simulink model "Citation"  (Simulink 10.0)
settings: Solver=ode5  StartTime=0.0  StopTime=700  FixedStep=0.01  RelTol=1e-3  EnableMultiTasking=on
values from neighbouring files (symbols this model uses):
  x0 = []    [cessnac550_3d_sfnc.m]
undefined symbols (not defined in the file or in its folder): chord, cv1, cv2, cv3, cv4, deltagmax1, deltagmax2, deltagmax3, deltagmax4, Deng, ealphag, ealphas, g0, hDME, hGS, kt1, kt2, kt3, lh, massinit, matbuaf, matdaf, matdam, matdbbf, matdeaf, matdgaf, matdqaf, matduaf, matdwaw, matedhr, mateif, matelhr, matemhr, matemv1, matemv2, matemve, matetam, mateuaf, matfaaf, matfaxl, matff, matibaf, matibmh, matipaf, matipmh, matiraf, matiuaf, matiwaf, matlaf, matlam, matleaf, matleam, matlgaf, matlqaf, matluaf, matmaaf, matmaam, matmaf, matmam, matmbbf ... (+77)
undefined symbols (not defined in the file): matibb
libraries: simulink x8, vrlib x1
(part 5 of 5)

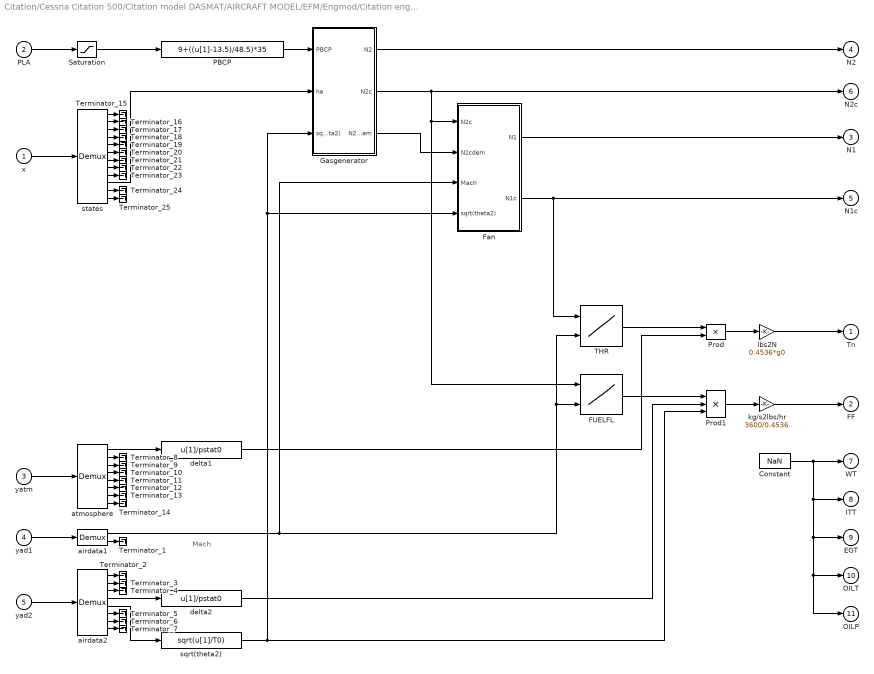
== system Citation/Cessna Citation 500/Citation model DASMAT/AIRCRAFT MODEL/EFM/Engmod/Citation eng_mod/Subsystem1/JT15 Dynamic1/Subsystem/engine ==
  note: Mach
  x : Inport
  PLA : Inport  Port=2
  yatm : Inport  Port=3
  yad1 : Inport  Port=4
  yad2 : Inport  Port=5
  Constant : Constant  Value=NaN
  FUELFL : Lookup2D  RowIndex=matff(2:14,1)  ColumnIndex=matff(1,2:14)  Table=matff(2:14,2:14)  SaturateOnIntegerOverflow=on  InputSameDT=on
  Fan : Subsystem
  Gasgenerator : Subsystem
  PBCP : Fcn  Expr=9+((u[1]-13.5)/48.5)*35
  Prod : Product  SaturateOnIntegerOverflow=on  InputSameDT=on  OutDataTypeStr=Inherit: Same as first input
  Prod1 : Product  Inputs=3  SaturateOnIntegerOverflow=on  InputSameDT=on  OutDataTypeStr=Inherit: Same as first input
  Saturation : Saturate  UpperLimit=62  LowerLimit=13.5
  THR : Lookup2D  RowIndex=matthr(2:12,1)  ColumnIndex=matthr(1,2:12)  Table=matthr(2:12,2:12)  SaturateOnIntegerOverflow=on  InputSameDT=on
  Terminator_{1..25} (25 alike) : Terminator
  airdata1 : Demux  Outputs=2
  airdata2 : Demux  Outputs=8
  atmosphere : Demux  Outputs=8
  delta1 : Fcn  Expr=u[1]/pstat0
  delta2 : Fcn  Expr=u[1]/pstat0
  kg/s2lbs/hr : Gain  Gain=3600/0.4536  SaturateOnIntegerOverflow=on  OutDataTypeStr=Inherit: Same as input  ParamDataTypeStr=Inherit: Same as input
  lbs2N : Gain  Gain=0.4536*g0  SaturateOnIntegerOverflow=on  OutDataTypeStr=Inherit: Same as input  ParamDataTypeStr=Inherit: Same as input
  sqrt(theta2) : Fcn  Expr=sqrt(u[1]/T0)
  states : Demux  Outputs=12
  Tn : Outport
  FF : Outport  Port=2
  N1 : Outport  Port=3
  N2 : Outport  Port=4
  N1c : Outport  Port=5
  N2c : Outport  Port=6
  WT : Outport  Port=7
  ITT : Outport  Port=8
  EGT : Outport  Port=9
  OILT : Outport  Port=10
  OILP : Outport  Port=11
  wires:
  states/12 -> Terminator_25/1
  states/11 -> Terminator_24/1
  states/9 -> Terminator_23/1
  states/8 -> Terminator_22/1
  states/7 -> Terminator_21/1
  states/6 -> Terminator_20/1
  states/5 -> Terminator_19/1
  states/4 -> Terminator_18/1
  states/3 -> Terminator_17/1
  states/2 -> Terminator_16/1
  states/1 -> Terminator_15/1
  atmosphere/8 -> Terminator_14/1
  atmosphere/7 -> Terminator_13/1
  atmosphere/6 -> Terminator_12/1
  atmosphere/5 -> Terminator_11/1
  atmosphere/4 -> Terminator_10/1
  atmosphere/3 -> Terminator_9/1
  atmosphere/2 -> Terminator_8/1
  airdata2/8 -> Terminator_7/1
  airdata2/7 -> Terminator_6/1
  airdata2/6 -> Terminator_5/1
  airdata2/3 -> Terminator_4/1
  airdata2/2 -> Terminator_3/1
  airdata2/1 -> Terminator_2/1
  airdata1/2 -> Terminator_1/1
  Fan/2(N1c) -> THR/1, N1c/1
  Gasgenerator/2(N2c) -> Fan/1(N2c), FUELFL/1, N2c/1
  Gasgenerator/3(N2cdem) -> Fan/2(N2cdem)
  airdata1/1 -> Fan/3(Mach), FUELFL/2, THR/2
  Fan/1(N1) -> N1/1
  sqrt(theta2)/1 -> Fan/4(sqrt(theta2)), Gasgenerator/3(sqrt(theta2)), Prod1/3
  yad2/1 -> airdata2/1
  yad1/1 -> airdata1/1
  yatm/1 -> atmosphere/1
  airdata2/4 -> delta2/1
  airdata2/5 -> sqrt(theta2)/1
  Constant/1 -> ITT/1, EGT/1, OILT/1, OILP/1, WT/1
  Gasgenerator/1(N2) -> N2/1
  delta1/1 -> Prod/2
  Prod/1 -> lbs2N/1
  THR/1 -> Prod/1
  lbs2N/1 -> Tn/1
  states/10 -> Gasgenerator/2(he)
  delta2/1 -> Prod1/2
  atmosphere/1 -> delta1/1
  Prod1/1 -> kg/s2lbs/hr/1
  kg/s2lbs/hr/1 -> FF/1
  Saturation/1 -> PBCP/1
  PLA/1 -> Saturation/1
  x/1 -> states/1
  PBCP/1 -> Gasgenerator/1(PBCP)
  FUELFL/1 -> Prod1/1

== system Citation/Cessna Citation 500/Citation model DASMAT/AIRCRAFT MODEL/EFM/Engmod/Citation eng_mod/Subsystem1/JT15 Dynamic/Subsystem/engine/Fan ==
  note: N1c feedback
  note: N1cdot
  N2c : Inport
  N2cdem : Inport  Port=2
  Mach : Inport  Port=3
  sqrt(theta2) : Inport  Port=4
  Droop : Gain  Gain=2  SaturateOnIntegerOverflow=on  OutDataTypeStr=Inherit: Same as input  ParamDataTypeStr=Inherit: Same as input
  Max accel : Subsystem  mask(Min Value){}
      mask help:
      | Output is minimum value of inputs.
      | y=min(u1,u2)
      mask Help: The Min block produces as output the minimum value of two scalars or vectors. If the inputs are vectors, the output will be a vector containing the minimum elements of the vectors.
      mask Display: disp('Min')
  Max decel : Subsystem  mask(Max Value){}
      mask help:
      | Output is maximum value of inputs.
      | y=max(u1,u2)
      mask Help: The Max block produces as output the maximum value of two scalars or vectors. If the inputs are vectors, the output will be a vector containing the maximum elements of the vectors.
      mask Display: disp('Max')
  N1 state : Integrator  InitialCondition=xt0(2)
  N1D : Lookup2D  RowIndex=matn1d(2:14,1)  ColumnIndex=matn1d(1,2:14)  Table=matn1d(2:14,2:14)  SaturateOnIntegerOverflow=on  InputSameDT=on
  Prod : Product  SaturateOnIntegerOverflow=on  InputSameDT=on  OutDataTypeStr=Inherit: Same as first input
  Sum : Sum  Inputs=+-  SaturateOnIntegerOverflow=on  InputSameDT=on  OutDataTypeStr=Inherit: Same as first input
  fN1cmax : Lookup  InputValues="[0 25 40 70 94  120]"  Table="[0   0   1   12 14  18]"  SaturateOnIntegerOverflow=on
  fN1cmin : Lookup  InputValues="[25     50   60   94 100]"  Table="[-0.05  -0.05    -1    -30 -28]"  SaturateOnIntegerOverflow=on
  N1 : Outport
  N1c : Outport  Port=2
  wires:
  sqrt(theta2)/1 -> Prod/2
  N1 state/1 -> Prod/1, Sum/2, N1c/1
  N2c/1 -> fN1cmin/1, fN1cmax/1
  Max decel/1(out_1) -> N1 state/1
  N1D/1 -> Sum/1
  Max accel/1(out_1) -> Max decel/1(in_1)
  fN1cmax/1 -> Max accel/2(in_2)
  fN1cmin/1 -> Max decel/2(in_2)
  Sum/1 -> Droop/1
  Droop/1 -> Max accel/1(in_1)
  Mach/1 -> N1D/2
  Prod/1 -> N1/1
  N2cdem/1 -> N1D/1

== system Citation/Cessna Citation 500/Citation model DASMAT/AIRCRAFT MODEL/EFM/Engmod/Citation eng_mod/Subsystem1/JT15 Dynamic/Subsystem/engine/Gasgenerator ==
  note: N2 feedback
  note: N2dot
  PBCP : Inport
  he : Inport  Port=2
  sqrt(theta2) : Inport  Port=3
  Droop : Lookup  InputValues=[0 100]  Table="[0.1  2]"  SaturateOnIntegerOverflow=on
  Fcn : Fcn  Expr=u[1]/u[2]
  Fcn1 : Fcn  Expr=u[1]/u[2]
  Governor : Product  SaturateOnIntegerOverflow=on  InputSameDT=on  OutDataTypeStr=Inherit: Same as first input
  Max accel : Subsystem  mask(Max Value){}
      mask help:
      | Output is maximum value of inputs.
      | y=max(u1,u2)
      mask Help: The Max block produces as output the maximum value of two scalars or vectors. If the inputs are vectors, the output will be a vector containing the maximum elements of the vectors.
      mask Display: disp('Max')
  Min accel : Subsystem  mask(Min Value){}
      mask help:
      | Output is minimum value of inputs.
      | y=min(u1,u2)
      mask Help: The Min block produces as output the minimum value of two scalars or vectors. If the inputs are vectors, the output will be a vector containing the minimum elements of the vectors.
      mask Display: disp('Min')
  Mux : Mux  Inputs=2
  Mux1 : Mux  Inputs=2
  N2 state : Integrator  InitialCondition=xt0(1)
  N2D : Lookup2D  RowIndex=matn2d(2:10,1)  ColumnIndex=matn2d(1,2:10)  Table=matn2d(2:10,2:10)  SaturateOnIntegerOverflow=on  InputSameDT=on
  Sum : Sum  Inputs=+-  SaturateOnIntegerOverflow=on  InputSameDT=on  OutDataTypeStr=Inherit: Same as first input
  fN2max : Lookup  InputValues=[25 40 70 94]  Table=[0 3 8 10]  SaturateOnIntegerOverflow=on
  fN2min : Lookup  InputValues="[25     50   60   94 100]"  Table="[-0.05  -0.05    -2    -20 -28]"  SaturateOnIntegerOverflow=on
  ft2FL : Gain  Gain=.01  SaturateOnIntegerOverflow=on  OutDataTypeStr=Inherit: Same as input  ParamDataTypeStr=Inherit: Same as input
  m2ft : Gain  Gain=(1/0.3048)  SaturateOnIntegerOverflow=on  OutDataTypeStr=Inherit: Same as input  ParamDataTypeStr=Inherit: Same as input
  N2 : Outport
  N2c : Outport  Port=2
  N2cdem : Outport  Port=3
  wires:
  sqrt(theta2)/1 -> Mux1/2, Mux/2
  N2D/1 -> Mux/1, Droop/1, Sum/1
  Fcn1/1 -> N2c/1
  Fcn/1 -> N2cdem/1
  Mux1/1 -> Fcn1/1
  Mux/1 -> Fcn/1
  Min accel/1(out_1) -> Max accel/1(in_1)
  ft2FL/1 -> N2D/2
  m2ft/1 -> ft2FL/1
  he/1 -> m2ft/1
  N2 state/1 -> Mux1/1, fN2min/1, fN2max/1, Sum/2, N2/1
  fN2max/1 -> Min accel/2(in_2)
  fN2min/1 -> Max accel/2(in_2)
  PBCP/1 -> N2D/1
  Droop/1 -> Governor/1
  Sum/1 -> Governor/2
  Governor/1 -> Min accel/1(in_1)
  Max accel/1(out_1) -> N2 state/1

== system Citation/Cessna Citation 500/Citation model DASMAT/AIRCRAFT MODEL/EFM/Engmod/Citation eng_mod/Subsystem1/JT15 Dynamic1/Subsystem/engine/Fan ==
  note: N1c feedback
  note: N1cdot
  N2c : Inport
  N2cdem : Inport  Port=2
  Mach : Inport  Port=3
  sqrt(theta2) : Inport  Port=4
  Droop : Gain  Gain=2  SaturateOnIntegerOverflow=on  OutDataTypeStr=Inherit: Same as input  ParamDataTypeStr=Inherit: Same as input
  Max accel : Subsystem  mask(Min Value){}
      mask help:
      | Output is minimum value of inputs.
      | y=min(u1,u2)
      mask Help: The Min block produces as output the minimum value of two scalars or vectors. If the inputs are vectors, the output will be a vector containing the minimum elements of the vectors.
      mask Display: disp('Min')
  Max decel : Subsystem  mask(Max Value){}
      mask help:
      | Output is maximum value of inputs.
      | y=max(u1,u2)
      mask Help: The Max block produces as output the maximum value of two scalars or vectors. If the inputs are vectors, the output will be a vector containing the maximum elements of the vectors.
      mask Display: disp('Max')
  N1 state : Integrator  InitialCondition=xt0(2)
  N1D : Lookup2D  RowIndex=matn1d(2:14,1)  ColumnIndex=matn1d(1,2:14)  Table=matn1d(2:14,2:14)  SaturateOnIntegerOverflow=on  InputSameDT=on
  Prod : Product  SaturateOnIntegerOverflow=on  InputSameDT=on  OutDataTypeStr=Inherit: Same as first input
  Sum : Sum  Inputs=+-  SaturateOnIntegerOverflow=on  InputSameDT=on  OutDataTypeStr=Inherit: Same as first input
  fN1cmax : Lookup  InputValues="[0 25 40 70 94  120]"  Table="[0   0   1   12 14  18]"  SaturateOnIntegerOverflow=on
  fN1cmin : Lookup  InputValues="[25     50   60   94 100]"  Table="[-0.05  -0.05    -1    -30 -28]"  SaturateOnIntegerOverflow=on
  N1 : Outport
  N1c : Outport  Port=2
  wires:
  sqrt(theta2)/1 -> Prod/2
  N1 state/1 -> Prod/1, Sum/2, N1c/1
  N2c/1 -> fN1cmin/1, fN1cmax/1
  Max decel/1(out_1) -> N1 state/1
  N1D/1 -> Sum/1
  Max accel/1(out_1) -> Max decel/1(in_1)
  fN1cmax/1 -> Max accel/2(in_2)
  fN1cmin/1 -> Max decel/2(in_2)
  Sum/1 -> Droop/1
  Droop/1 -> Max accel/1(in_1)
  Mach/1 -> N1D/2
  Prod/1 -> N1/1
  N2cdem/1 -> N1D/1

== system Citation/Cessna Citation 500/Citation model DASMAT/AIRCRAFT MODEL/EFM/Engmod/Citation eng_mod/Subsystem1/JT15 Dynamic1/Subsystem/engine/Gasgenerator ==
  note: N2 feedback
  note: N2dot
  PBCP : Inport
  he : Inport  Port=2
  sqrt(theta2) : Inport  Port=3
  Droop : Lookup  InputValues=[0 100]  Table="[0.1  2]"  SaturateOnIntegerOverflow=on
  Fcn : Fcn  Expr=u[1]/u[2]
  Fcn1 : Fcn  Expr=u[1]/u[2]
  Governor : Product  SaturateOnIntegerOverflow=on  InputSameDT=on  OutDataTypeStr=Inherit: Same as first input
  Max accel : Subsystem  mask(Max Value){}
      mask help:
      | Output is maximum value of inputs.
      | y=max(u1,u2)
      mask Help: The Max block produces as output the maximum value of two scalars or vectors. If the inputs are vectors, the output will be a vector containing the maximum elements of the vectors.
      mask Display: disp('Max')
  Min accel : Subsystem  mask(Min Value){}
      mask help:
      | Output is minimum value of inputs.
      | y=min(u1,u2)
      mask Help: The Min block produces as output the minimum value of two scalars or vectors. If the inputs are vectors, the output will be a vector containing the minimum elements of the vectors.
      mask Display: disp('Min')
  Mux : Mux  Inputs=2
  Mux1 : Mux  Inputs=2
  N2 state : Integrator  InitialCondition=xt0(1)
  N2D : Lookup2D  RowIndex=matn2d(2:10,1)  ColumnIndex=matn2d(1,2:10)  Table=matn2d(2:10,2:10)  SaturateOnIntegerOverflow=on  InputSameDT=on
  Sum : Sum  Inputs=+-  SaturateOnIntegerOverflow=on  InputSameDT=on  OutDataTypeStr=Inherit: Same as first input
  fN2max : Lookup  InputValues=[25 40 70 94]  Table=[0 3 8 10]  SaturateOnIntegerOverflow=on
  fN2min : Lookup  InputValues="[25     50   60   94 100]"  Table="[-0.05  -0.05    -2    -20 -28]"  SaturateOnIntegerOverflow=on
  ft2FL : Gain  Gain=.01  SaturateOnIntegerOverflow=on  OutDataTypeStr=Inherit: Same as input  ParamDataTypeStr=Inherit: Same as input
  m2ft : Gain  Gain=(1/0.3048)  SaturateOnIntegerOverflow=on  OutDataTypeStr=Inherit: Same as input  ParamDataTypeStr=Inherit: Same as input
  N2 : Outport
  N2c : Outport  Port=2
  N2cdem : Outport  Port=3
  wires:
  sqrt(theta2)/1 -> Mux1/2, Mux/2
  N2D/1 -> Mux/1, Droop/1, Sum/1
  Fcn1/1 -> N2c/1
  Fcn/1 -> N2cdem/1
  Mux1/1 -> Fcn1/1
  Mux/1 -> Fcn/1
  Min accel/1(out_1) -> Max accel/1(in_1)
  ft2FL/1 -> N2D/2
  m2ft/1 -> ft2FL/1
  he/1 -> m2ft/1
  N2 state/1 -> Mux1/1, fN2min/1, fN2max/1, Sum/2, N2/1
  fN2max/1 -> Min accel/2(in_2)
  fN2min/1 -> Max accel/2(in_2)
  PBCP/1 -> N2D/1
  Droop/1 -> Governor/1
  Sum/1 -> Governor/2
  Governor/1 -> Min accel/1(in_1)
  Max accel/1(out_1) -> N2 state/1

== system Citation/Cessna Citation 500/Citation model DASMAT/AIRCRAFT MODEL/EFM/Engmod/Citation eng_mod/Subsystem1/JT15 Dynamic/Subsystem/engine/Fan/Max accel ==
  in_1 : Inport
  in_2 : Inport  Port=2
  Sum : Sum  Inputs=-+  SaturateOnIntegerOverflow=on  InputSameDT=on  OutDataTypeStr=Inherit: Same as first input
  Switch : Switch  SaturateOnIntegerOverflow=on  InputSameDT=on
  out_1 : Outport
  wires:
  in_1/1 -> Sum/1, Switch/1
  in_2/1 -> Sum/2, Switch/3
  Sum/1 -> Switch/2
  Switch/1 -> out_1/1

== system Citation/Cessna Citation 500/Citation model DASMAT/AIRCRAFT MODEL/EFM/Engmod/Citation eng_mod/Subsystem1/JT15 Dynamic/Subsystem/engine/Fan/Max decel ==
  in_1 : Inport
  in_2 : Inport  Port=2
  Sum : Sum  Inputs=+-  SaturateOnIntegerOverflow=on  InputSameDT=on  OutDataTypeStr=Inherit: Same as first input
  Switch : Switch  SaturateOnIntegerOverflow=on  InputSameDT=on
  out_1 : Outport
  wires:
  Switch/1 -> out_1/1
  Sum/1 -> Switch/2
  in_2/1 -> Sum/2, Switch/3
  in_1/1 -> Sum/1, Switch/1

== system Citation/Cessna Citation 500/Citation model DASMAT/AIRCRAFT MODEL/EFM/Engmod/Citation eng_mod/Subsystem1/JT15 Dynamic/Subsystem/engine/Gasgenerator/Max accel ==
  in_1 : Inport
  in_2 : Inport  Port=2
  Sum : Sum  Inputs=+-  SaturateOnIntegerOverflow=on  InputSameDT=on  OutDataTypeStr=Inherit: Same as first input
  Switch : Switch  SaturateOnIntegerOverflow=on  InputSameDT=on
  out_1 : Outport
  wires:
  Switch/1 -> out_1/1
  Sum/1 -> Switch/2
  in_2/1 -> Sum/2, Switch/3
  in_1/1 -> Sum/1, Switch/1

== system Citation/Cessna Citation 500/Citation model DASMAT/AIRCRAFT MODEL/EFM/Engmod/Citation eng_mod/Subsystem1/JT15 Dynamic/Subsystem/engine/Gasgenerator/Min accel ==
  in_1 : Inport
  in_2 : Inport  Port=2
  Sum : Sum  Inputs=-+  SaturateOnIntegerOverflow=on  InputSameDT=on  OutDataTypeStr=Inherit: Same as first input
  Switch : Switch  SaturateOnIntegerOverflow=on  InputSameDT=on
  out_1 : Outport
  wires:
  in_1/1 -> Sum/1, Switch/1
  in_2/1 -> Sum/2, Switch/3
  Sum/1 -> Switch/2
  Switch/1 -> out_1/1

== system Citation/Cessna Citation 500/Citation model DASMAT/AIRCRAFT MODEL/EFM/Engmod/Citation eng_mod/Subsystem1/JT15 Dynamic1/Subsystem/engine/Fan/Max accel ==
  in_1 : Inport
  in_2 : Inport  Port=2
  Sum : Sum  Inputs=-+  SaturateOnIntegerOverflow=on  InputSameDT=on  OutDataTypeStr=Inherit: Same as first input
  Switch : Switch  SaturateOnIntegerOverflow=on  InputSameDT=on
  out_1 : Outport
  wires:
  in_1/1 -> Sum/1, Switch/1
  in_2/1 -> Sum/2, Switch/3
  Sum/1 -> Switch/2
  Switch/1 -> out_1/1

== system Citation/Cessna Citation 500/Citation model DASMAT/AIRCRAFT MODEL/EFM/Engmod/Citation eng_mod/Subsystem1/JT15 Dynamic1/Subsystem/engine/Fan/Max decel ==
  in_1 : Inport
  in_2 : Inport  Port=2
  Sum : Sum  Inputs=+-  SaturateOnIntegerOverflow=on  InputSameDT=on  OutDataTypeStr=Inherit: Same as first input
  Switch : Switch  SaturateOnIntegerOverflow=on  InputSameDT=on
  out_1 : Outport
  wires:
  Switch/1 -> out_1/1
  Sum/1 -> Switch/2
  in_2/1 -> Sum/2, Switch/3
  in_1/1 -> Sum/1, Switch/1

== system Citation/Cessna Citation 500/Citation model DASMAT/AIRCRAFT MODEL/EFM/Engmod/Citation eng_mod/Subsystem1/JT15 Dynamic1/Subsystem/engine/Gasgenerator/Max accel ==
  in_1 : Inport
  in_2 : Inport  Port=2
  Sum : Sum  Inputs=+-  SaturateOnIntegerOverflow=on  InputSameDT=on  OutDataTypeStr=Inherit: Same as first input
  Switch : Switch  SaturateOnIntegerOverflow=on  InputSameDT=on
  out_1 : Outport
  wires:
  Switch/1 -> out_1/1
  Sum/1 -> Switch/2
  in_2/1 -> Sum/2, Switch/3
  in_1/1 -> Sum/1, Switch/1

== system Citation/Cessna Citation 500/Citation model DASMAT/AIRCRAFT MODEL/EFM/Engmod/Citation eng_mod/Subsystem1/JT15 Dynamic1/Subsystem/engine/Gasgenerator/Min accel ==
  in_1 : Inport
  in_2 : Inport  Port=2
  Sum : Sum  Inputs=-+  SaturateOnIntegerOverflow=on  InputSameDT=on  OutDataTypeStr=Inherit: Same as first input
  Switch : Switch  SaturateOnIntegerOverflow=on  InputSameDT=on
  out_1 : Outport
  wires:
  in_1/1 -> Sum/1, Switch/1
  in_2/1 -> Sum/2, Switch/3
  Sum/1 -> Switch/2
  Switch/1 -> out_1/1

== matlab function Instrument Block/MATLAB Function ==
  data: phi input double; phi_r output double; theta input double; theta_r output double
function [phi_r, theta_r] = fcn(phi, theta)

phi_r = phi;
theta_r = theta;

if phi_r > 180
    phi_r = -180+(phi_r-180);
elseif phi_r < -180
    phi_r = 180+(phi_r+180);
end

== matlab function Flight Controllers/ANDI/ANDI/AMI w//Stat Method/Statistical Methods/Moving Average/Moving Average Function ==
  data: Delta_k input double; avg output double; n_k1 input double; data input double; n_k output double; data output double
function [avg, n_k, data] = movavg(Delta_k, n_k1, data)
offset = 1000; %[-] Start index of covariance computation
w = 25; %[-] Window Length

if n_k1 < offset - w
    n_k = n_k1+1;
    avg = nan(1,6);
 
elseif n_k1 >= offset - w && n_k1 < offset
    n_k = n_k1+1;
    data(n_k-offset+w,:) = Delta_k.^2;
    avg = nan(1,6);

elseif n_k1 >= offset
    n_k = n_k1+1;
    data(mod(n_k-1,w)+1,:) = Delta_k.^2;
    avg = mean(data);

else
    error('Moving Average Function Error')
end

== matlab function Flight Controllers/ANDI/ANDI/AMI w//Loss/Aerodynamic Coefficients ==
  data: x input double; y_k output double
function y_k  = aerocoeff(x)
% Constants
m = 4500; %[kg]

%% Aircraft Geometry

% Mass Moments of Inertia
Ixx = 11187.8; %[kg/m^2]
Iyy = 22854.8; %[kg/m^2]
Izz = 31974.8; %[kg/m^2]
Ixz = 1930.1; %[kg/m^2]

% Wing Geometry
b = 13.3250; %Wing Span [m]
S = 24.9900; %Wing Area [m^2]
c = 1.9910; %Chord Length [m]

%% Aircraft State
rho = x(15); %[kg/m^3]
Vtas = x(7); %[m/s]

% Angular Velocities
p = x(1);  %[rad/s]
q = x(2);  %[rad/s]
r = x(3);  %[rad/s]

% Angular Accelerations
pdot = x(4); %[rad/s^2]
qdot = x(5); %[rad/s^2]
rdot = x(6); %[rad/s^2]

% Linear Accelerations
xac = x(16); %[m/s^2]
yac = x(17); %[m/s^2]
zac = x(18); %[m/s^2]

%% Aerodynamic Coefficients
den = (0.5*rho*Vtas^2*S); 

% Force Coefficients
CX = (m*xac)/den;
CY = (m*yac)/den;
CZ = (m*zac)/den;

% Moment Coefficients
Cl = (pdot*Ixx + q*r*(Izz-Iyy) - (p*q+rdot)*Ixz)/(den*b);
Cm = (qdot*Iyy + r*p*(Ixx-Izz) + (p^2-r^2)*Ixz)/(den*c);
Cn = (rdot*Izz + p*q*(Iyy-Ixx) + (q*r-pdot)*Ixz)/(den*b);

y_k = [CX, CZ, Cm, CY, Cl, Cn];
end

== matlab function Flight Controllers/ANDI/ANDI/AMI w//Stat Method/Statistical Methods/Auto-Correlation/Auto-Correlation Function ==
  data: Delta_k input double; corr output double; data input double; n_k1 input double; data output double; n_k output double
function [corr, data, n_k] = auto_corr(Delta_k, data, n_k1)
N = 100; %[-] sample window length
ov = 50; %[-] overlap/buffer size


if n_k1 < N
    n_k = n_k1+1;
    data(n_k,:) = Delta_k;
    corr = zeros(1,6);
    
elseif n_k1 >= N
    d = zeros(2*N-1,6);
    for i = 1:6
        [c, lags] = xcorr(data(:,i), 'unbiased');
        d(:,i) = c;
    end
    
    corr = d(N+1,:);

    data = cat(1,data(1:ov,:),zeros(N-ov,6));
    n_k = ov;
else
    error('Correlation Function Error')
end

end

== matlab function Flight Controllers/ANDI/ANDI/AMI w//Loss/Inputs1 ==
  data: x input double; h_k output double
function h_k  = hcalc(x)
% Wing Geometry
b = 13.3250; %Wing Span [m]
c = 1.9910; %Chord Length [m]

% Angular Velocities
p = x(1);  %[rad/s]
q = x(2);  %[rad/s]
r = x(3);  %[rad/s]

% Aircraft States
Vtas = x(7); %[m/s]
alpha = x(8); %[rad]
beta = x(9); %[rad]

% Measured Deflections
de = x(19); %[rad]
da = x(20); %[rad]
dr = x(21); %[rad]

% Aircraft State Components
hX_k = [1; alpha; alpha^2; q*c/Vtas; de; 0];
hZ_k = [1; alpha; q*c/Vtas; de; 0; 0];
hm_k = [1; alpha; q*c/Vtas; de; 0; 0];

hY_k = [1; beta; p*b/(2*Vtas); r*b/(2*Vtas); da; dr];
hl_k = [1; beta; p*b/(2*Vtas); r*b/(2*Vtas); da; dr];
hn_k = [1; beta; p*b/(2*Vtas); r*b/(2*Vtas); da; dr];

h_k = [hX_k, hZ_k, hm_k, hY_k, hl_k, hn_k];
end

== matlab function State Vector/MATLAB Function1 ==
  settings: updateMethod=DISCRETE
  data: V input double; u output double; alpha input double; beta input double; v output double; w output double
%% AirSpeed Components Function
function [u, v, w] = AirspeedComp(V, alpha, beta)
u = V*cos(alpha)*cos(beta);
v = V*sin(beta);
w = V*sin(alpha);

== matlab function State Vector/MATLAB Function2 ==
  settings: updateMethod=DISCRETE
  data: h input double; rho output double
%% Air Density Function (DensCalc)
function rho = Denscalc(h)

% Atmospheric Coefficients
R = 287.05; %[m^2/K s^2]
g = 9.807; %[m/s^2]
T_0 = 288.15; %[K]
rho_0 = 1.225; %[kg/m^3]
lambda_trop = -0.0065; %[K/m]

% Atmospheric Layers
h_0 = 0; %[m]
h_trop = 11*1000; %[m]
h_strat = 20*1000; %[m]

% Calculating Constants
persistent T_trop rho_trop
if isempty(T_trop) || isempty(rho_trop)
    T_trop = T_0 + (h_trop - h_0)*lambda_trop; %[K]
    rho_trop = rho_0*(1 + lambda_trop*h_trop/T_0)^(-g/(R*lambda_trop) - 1); %[kg/m^3]
end

%rho_strato = rho_trop*exp(-g/(R*T_trop)*(h_strat - h_trop)); %[kg/m^3]

% Calculating Density
if h <= h_trop && h >= 0
    rho = rho_0*(1 + lambda_trop*h/T_0)^(-g/(R*lambda_trop) - 1); %[kg/m^3]
elseif h > h_trop && h <= h_strat
    rho = rho_trop*exp(-g/(R*T_trop)*(h - h_trop)); %[kg/m^3]
else 
    error('DensCalc Function Error. \nInvalid Altitude Range h = %d (0 <= h <= 20000) \n', h)
end

end

== matlab function Flight Controllers/Controller Switch/MATLAB Function ==
  data: input input double size=[4,1]; output output double size=[1,1] [1..4]; prev input double size=[1,1]
function output = cswtch(input, prev)
output = max(input);

if output == 0
    output = prev;   
end
end

== matlab function Flight Controllers/ANDI/ANDI/AMI w//Loss/Recursive Least Squares w//Loss ==
  data: y_k input double; h_k input double; pmat_k output double; pmat_k input double; Pmat_k input double; Pmat_k output double; Delta_k output double
function [pmat_k, Pmat_k, Delta_k] = RLSL(y_k, h_k, pmat_k, Pmat_k)
% Forgetting Factor Vector
lambda = 0.99*ones(1,6);

% Recursive Least Squares
for idx=1:length(y_k)
    rlsl(idx, y_k(idx), pmat_k(:,idx), Pmat_k(:,6*idx-5:6*idx), h_k(:,idx));
end

function [p_k, P_k] = rlsl(idx, y_k, p_k1, P_k1, h_k)   
L_k = P_k1*h_k*(h_k.'*P_k1*h_k+lambda(idx))^-1;
p_k = p_k1 + L_k*(y_k - h_k.'*p_k1);
P_k = (eye(length(h_k))-L_k*h_k.')*P_k1/lambda(idx);

pmat_k(:,idx) = p_k;
Pmat_k(:,6*idx-5:6*idx) = P_k;
end

Delta_k = y_k - diag(h_k.'*pmat_k).';
end

== matlab function Flight Controllers/INDI/INDI/Dynamic Inversion B ==
  data: Y input double; x input double; dU output double
function dU = DynInvB(Y, x)
% Aircraft State
Vtas = x(7); %[m/s]
rho = x(15); %[kg/m^3]

% Wing Geometry
S = 24.9900; %Wing Area [m^2]
b = 13.3250; %Wing Span [m]
c = 1.9910; %Chord Length [m]

dyn = 0.5*rho*Vtas^2*S; % [N/m]

% Mass Moments of Inertia
Ixx = 11187.8; %[kg/m^2]
Iyy = 22854.8; %[kg/m^2]
Izz = 31974.8; %[kg/m^2]
Ixz = 1930.1; %[kg/m^2]
I = [Ixx, 0, -Ixz; 0, Iyy, 0; -Ixz, 0, Izz];

% Aerodynamic Coefficients
Clda = -0.184;
Cldr = 0.034;
Cmde = -0.894;
Cnda = -0.011;
Cndr = -0.097;

C = [b*Clda, 0, b*Cldr; 0, c*Cmde, 0; b*Cnda, 0, b*Cndr];

dU = C\((I/dyn)*Y);

== matlab function Flight Controllers/INDI/INDI/Kynematic Inversion A ==
  data: x input double; a output double
function a = KynInvA(x)
% Constants 
g = 9.807; %[m/s^2]

% Aircraft States
V = x(7); %[m/s]
phi = x(13); %[rad]
theta = x(14); %[rad]

% Airspeed Components
u = x(10);  %[m/s]
v = x(11);  %[m/s]
w = x(12);  %[m/s]

% Linear Accelerations
xac = x(16); %[m/s^2]
yac = x(17); %[m/s^2]
zac = x(18); %[m/s^2]

ax = xac - g*sin(theta);
ay = yac + g*sin(phi)*cos(theta);
az = zac + g*cos(phi)*cos(theta);

a = -[0; 0; (1/sqrt(u^2+w^2))*(-u*v*ax/V^2 + (1 - v/V^2)*ay - v*w*az/V^2)];

== matlab function Flight Controllers/INDI/INDI/Kynematic Inversion B ==
  data: Y input double; x input double; U output double
function U = KynInvB(Y, x)
% Aircraft States
phi = x(13); %[rad]
theta = x(14); %[rad]

% Airspeed Components
u = x(10);  %[m/s]
w = x(12);  %[m/s]

B = [1, sin(phi)*tan(theta), cos(phi)*tan(theta); 0, cos(phi), -sin(phi); ...
    w/sqrt(u^2+w^2), 0, -u/sqrt(u^2+w^2)];

U = B\Y;

== matlab function Flight Controllers/ANDI/ANDI/AMI w//Stat Method/Aerodynamic Coefficients ==
  data: x input double; y_k output double
function y_k  = aerocoeff(x)
% Constants
m = 4500; %[kg]

%% Aircraft Geometry

% Mass Moments of Inertia
Ixx = 11187.8; %[kg/m^2]
Iyy = 22854.8; %[kg/m^2]
Izz = 31974.8; %[kg/m^2]
Ixz = 1930.1; %[kg/m^2]

% Wing Geometry
b = 13.3250; %Wing Span [m]
S = 24.9900; %Wing Area [m^2]
c = 1.9910; %Chord Length [m]

%% Aircraft State
rho = x(15); %[kg/m^3]
Vtas = x(7); %[m/s]

% Angular Velocities
p = x(1);  %[rad/s]
q = x(2);  %[rad/s]
r = x(3);  %[rad/s]

% Angular Accelerations
pdot = x(4); %[rad/s^2]
qdot = x(5); %[rad/s^2]
rdot = x(6); %[rad/s^2]

% Linear Accelerations
xac = x(16); %[m/s^2]
yac = x(17); %[m/s^2]
zac = x(18); %[m/s^2]

%% Aerodynamic Coefficients
den = (0.5*rho*Vtas^2*S); 

% Force Coefficients
CX = (m*xac)/den;
CY = (m*yac)/den;
CZ = (m*zac)/den;

% Moment Coefficients
Cl = (pdot*Ixx + q*r*(Izz-Iyy) - (p*q+rdot)*Ixz)/(den*b);
Cm = (qdot*Iyy + r*p*(Ixx-Izz) + (p^2-r^2)*Ixz)/(den*c);
Cn = (rdot*Izz + p*q*(Iyy-Ixx) + (q*r-pdot)*Ixz)/(den*b);

y_k = [CX, CZ, Cm, CY, Cl, Cn];
end

== matlab function Flight Controllers/ANDI/ANDI/AMI w//Stat Method/Inputs ==
  data: x input double; h_k output double
function h_k  = hcalc(x)
% Wing Geometry
b = 13.3250; %Wing Span [m]
c = 1.9910; %Chord Length [m]

% Angular Velocities
p = x(1);  %[rad/s]
q = x(2);  %[rad/s]
r = x(3);  %[rad/s]

% Aircraft States
Vtas = x(7); %[m/s]
alpha = x(8); %[rad]
beta = x(9); %[rad]

% Measured Deflections
de = x(19); %[rad]
da = x(20); %[rad]
dr = x(21); %[rad]

% Aircraft State Components
hX_k = [1; alpha; alpha^2; q*c/Vtas; de; 0];
hZ_k = [1; alpha; q*c/Vtas; de; 0; 0];
hm_k = [1; alpha; q*c/Vtas; de; 0; 0];

hY_k = [1; beta; p*b/(2*Vtas); r*b/(2*Vtas); da; dr];
hl_k = [1; beta; p*b/(2*Vtas); r*b/(2*Vtas); da; dr];
hn_k = [1; beta; p*b/(2*Vtas); r*b/(2*Vtas); da; dr];

h_k = [hX_k, hZ_k, hm_k, hY_k, hl_k, hn_k];
end

== matlab function Flight Controllers/ANDI/ANDI/AMI w//Stat Method/Recursive Least Squares ==
  data: y_k input double; h_k input double; pmat_k output double; pmat_k input double; Pmat_k input double; Pmat_k output double; Delta_k output double; reset input double
function [pmat_k, Pmat_k, Delta_k] = RLS(y_k, h_k, pmat_k, Pmat_k, reset)
% Resetting the Covariance Matrix
for x = 1:length(reset)
    if reset(x) == 1
        Pmat_k(:,6*x-5:6*x) = diag(10000*ones(1,6));
    end
end

% Recursive Least Squares
for idx = 1:length(y_k)
    rls(idx, y_k(idx), pmat_k(:,idx), Pmat_k(:,6*idx-5:6*idx), h_k(:,idx));
end

function [p_k, P_k] = rls(idx, y_k, p_k1, P_k1, h_k)   
L_k = P_k1*h_k*(h_k.'*P_k1*h_k+1)^-1;
p_k = p_k1 + L_k*(y_k - h_k.'*p_k1);
P_k = (eye(length(h_k))-L_k*h_k.')*P_k1;

pmat_k(:,idx) = p_k;
Pmat_k(:,6*idx-5:6*idx) = P_k;
end

Delta_k = y_k - diag(h_k.'*pmat_k).';
end

== matlab function Flight Controllers/ANDI/ANDI/AMI w//Stat Method/Statistical Methods/MATLAB Function ==
  data: avg input double; reset output double; n_k1 input double; n_k output double
function [reset, n_k] = reset(avg, n_k1)
uppperlim =  [1, 0.1, 1, 0.1, 1e-4, 1e-4];
graceprd = 1000;

n_k = n_k1.' + 1;
A = avg > uppperlim;

if sum(A(1:3)) > 0 && sum(A(4:6)) > 0 && n_k(1) >= graceprd && ...
    n_k(2) >= graceprd && n_k(3) >= graceprd
    reset = ones(1,6);
    n_k(1) = 0;
elseif sum(A(1:3)) > 0 && n_k(1) >= graceprd && n_k(2) >= graceprd
    reset = [1 1 1 0 0 0];
    n_k(2) = 0;
elseif sum(A(4:6)) > 0 && n_k(1) >= graceprd && n_k(3) >= graceprd
    reset = [0 0 0 1 1 1];
    n_k(3) = 0;
else 
    reset = zeros(1,6);
end

== matlab function Flight Controllers/ANDI/ANDI/AMI w//Stat Method/Statistical Methods/Variance/Variance Function ==
  data: Delta_k input double; var output double; n_k1 input double; sm_k1 input double; smsq_k1 input double; n_k output double; sm_k output double; smsq_k output double
function [var, n_k, sm_k, smsq_k] = varcalc(Delta_k, n_k1, sm_k1, smsq_k1)
offset = 1000; %[-] Start index of covariance computation
ov = 200;

if n_k1 < offset-ov
    sm_k = zeros(1,6);
    smsq_k = zeros(1,6);
    n_k = n_k1+1;
    var = nan(1,6);
    
elseif n_k1 >= offset-ov && n_k1 < offset
    sm_k = sm_k1.' + Delta_k;
    smsq_k = smsq_k1.' + Delta_k.^2;
    n_k = n_k1+1;
    var = nan(1,6);
 
elseif n_k1 >= offset
    sm_k = sm_k1.' + Delta_k;
    smsq_k = smsq_k1.' + Delta_k.^2;
    n_k = n_k1+1;
    n = n_k - offset + ov;
    var = (smsq_k - (sm_k.^2)/n)/(n-1);
    
else
    error('Variance Function Error')
end

== matlab function Flight Controllers/ANDI/ANDI/AMI w//Stat Method/Statistical Methods/Whiteness Test/Whiteness Test Function ==
  data: Delta_k input double; test output double; data input double; n_k1 input double; data output double; n_k output double
function [test, data, n_k] = whitetest(Delta_k, data, n_k1)
N = 200; %[-] sample window length
ov = 50; %[-] overlap/buffer size

%Testing
k = 30; %[-] test window length
p = 5; %[-]

plotting = false;


if n_k1 < N
    n_k = n_k1+1;
    data(n_k,:) = Delta_k;
    test = zeros(1,13);
    
elseif n_k1 >= N
    corr = zeros(2*N-1,6);
    for i = 1:6
        [c, lags] = xcorr(data(:,i), 'unbiased');
        corr(:,i) = c;
    end

    w = matdiv(N*corr.^2, corr(N,:).^2);
   
    if plotting == true
        figure(1)
        plot(lags, corr);
        
        figure(2)
        plot(lags, w);
    end
    
    
    % Test 1
    cond1 = 1.95*corr(N,:)/sqrt(N);
    G = zeros(k,6);
    for x = 1:k
        g = corr(N+x,:) <= cond1;
        G(x,:) = g;
    end
    test1 = sum(G) >= (k-p)*ones(1,6);
    
    % Test 2
    cond2 = (k+1.65*sqrt(2*k))*(1/N)*corr(N,:).^2;
    sm = sum(corr(N+1:N+k+1,:).^2);
    test2 = sm <= cond2;
    
    test = [1, test1, test2];

    data = cat(1,data(1:ov,:),zeros(N-ov,6));
    n_k = ov;
else
    error('Correlation Function Error')
end

function C = matdiv(A,B)
    B = B.^(-1);
    C = A*diag(B);
    C(isnan(C)) = 0;
end

end

== matlab function Flight Controllers/ANDI/ANDI/Dynamic Inversion A ==
  data: x input double; a output double; p_k input double
function a = DynInvA(x, p_k)
% Aircraft States
Vtas = x(7); %[m/s]
alpha = x(8); %[rad]
beta = x(9); %[rad]
rho = x(15); %[kg/m^3]

% Wing Geometry
S = 24.9900; %Wing Area [m^2]
b = 13.3250; %Wing Span [m]
c = 1.9910; %Chord Length [m]

dyn = 0.5*rho*Vtas^2*S; % [N/m]

% Angular Velocities
p = x(1);  %[rad/s]
q = x(2);  %[rad/s]
r = x(3);  %[rad/s]
omega = [p; q; r];

% Mass Moments of Inertia
Ixx = 11187.8; %[kg/m^2]
Iyy = 22854.8; %[kg/m^2]
Izz = 31974.8; %[kg/m^2]
Ixz = 1930.1; %[kg/m^2]
I = [Ixx, 0, -Ixz; 0, Iyy, 0; -Ixz, 0, Izz];

Cla = dot([1; beta; p*b/(2*Vtas); r*b/(2*Vtas)], p_k(1:4,5));
Cma = dot([1; alpha; q*c/Vtas], p_k(1:3,3));
Cna = dot([1; beta; p*b/(2*Vtas); r*b/(2*Vtas)], p_k(1:4,6));
Ca = [b*Cla; c*Cma; b*Cna];

a = -inv(I)*(cross(omega,I*omega)-dyn*Ca);

== matlab function Flight Controllers/ANDI/ANDI/Dynamic Inversion B ==
  data: Y input double; x input double; U output double; p_k input double
function U = DynInvB(Y, x, p_k)
% Aircraft State
Vtas = x(7); %[m/s]
rho = x(15); %[kg/m^3]

% Wing Geometry
S = 24.9900; %Wing Area [m^2]
b = 13.3250; %Wing Span [m]
c = 1.9910; %Chord Length [m]

dyn = 0.5*rho*Vtas^2*S; % [N/m]

% Mass Moments of Inertia
Ixx = 11187.8; %[kg/m^2]
Iyy = 22854.8; %[kg/m^2]
Izz = 31974.8; %[kg/m^2]
Ixz = 1930.1; %[kg/m^2]
I = [Ixx, 0, -Ixz; 0, Iyy, 0; -Ixz, 0, Izz];

C = [b*p_k(5,5), 0, b*p_k(6,5); 0, c*p_k(4,3), 0; b*p_k(5,6), 0, b*p_k(6,6)];

U = C\((I/dyn)*Y);

== matlab function Flight Controllers/ANDI/ANDI/Kynematic Inversion A ==
  data: x input double; a output double
function a = KynInvA(x)
% Constants 
g = 9.807; %[m/s^2]

% Aircraft States
V = x(7); %[m/s]
phi = x(13); %[rad]
theta = x(14); %[rad]

% Airspeed Components
u = x(10);  %[m/s]
v = x(11);  %[m/s]
w = x(12);  %[m/s]

% Linear Accelerations
xac = x(16); %[m/s^2]
yac = x(17); %[m/s^2]
zac = x(18); %[m/s^2]

ax = xac - g*sin(theta);
ay = yac + g*sin(phi)*cos(theta);
az = zac + g*cos(phi)*cos(theta);

a = [0; 0; -(1/sqrt(u^2+w^2))*(-u*v*ax/V^2 + (1 - v/V^2)*ay - v*w*az/V^2)];

== matlab function Flight Controllers/ANDI/ANDI/Kynematic Inversion B ==
  data: Y input double; x input double; U output double
function U = KynInvB(Y, x)
% Aircraft States
phi = x(13); %[rad]
theta = x(14); %[rad]

% Airspeed Components
u = x(10);  %[m/s]
w = x(12);  %[m/s]

B = [1, 0, 0; 0, 1, 0; ...
    w/sqrt(u^2+w^2), 0, -u/sqrt(u^2+w^2)];

U = B\Y;
